simulink model "WriteToServo_test"  (R2014b)
settings: Solver=ode3  StartTime=0.0  StopTime=60  RelTol=1e-3
libraries: ServoCommand x2, BeagleBoneBlackCom x1
settings Model: SimulationMode=external  Creator=Sebastian  LastModifiedBy=Sebastian
settings OptimizationCC: OptimizeModelRefInitCode=on  LifeSpan=1  MaxStackSize=64
settings HardwareCC: ProdLargestAtomicInteger=Long  ProdLargestAtomicFloat=Double  ProdEndianess=LittleEndian  ProdHWDeviceType=ARM Compatible->ARM Cortex
settings RTWCC: SystemTargetFile=ert.tlc  TLCOptions=-aInlineSetEventsForThisBaseRateFcn=TLC_FALSE -aSuppressMultiTaskScheduler=TLC_FALSE  TemplateMakefile=ert_default_tmf  Description=Embedded Coder  ProcessScript=ert_make_rtw_hook  Toolchain=Linaro Toolchain v4.8  BuildConfiguration=Specify
settings CodeAppCC: IgnoreCustomStorageClasses=off

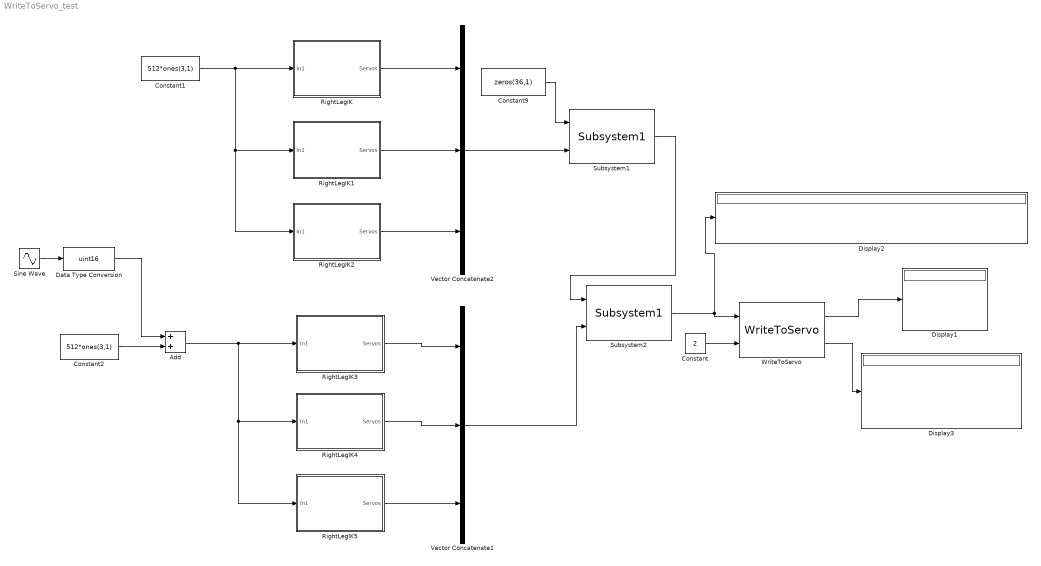
== system WriteToServo_test ==
  Add : Sum
  Constant : Constant  Value=2  OutDataTypeStr=uint8
  Constant1 : Constant  Value=512*ones(3,1)  OutDataTypeStr=uint16  SampleTime=-1
  Constant2 : Constant  Value=512*ones(3,1)  OutDataTypeStr=uint16  SampleTime=-1
  Constant9 : Constant  Value=zeros(36,1)  OutDataTypeStr=uint8  SampleTime=-1
  Data Type Conversion : DataTypeConversion  OutDataTypeStr=uint16
  Display1 : Display
      settings: Format=hex (Stored Integer)
  Display2 : Display
      settings: Format=hex (Stored Integer)
  Display3 : Display
      settings: Format=hex (Stored Integer)
  RightLegIK : Subsystem  TreatAsAtomicUnit=on  RTWFcnName=RightLegIK  mask{ID1=1, ID2=2, ID3=3}
      mask prompts: ID1 "Id servo 1"; ID2 "Id servo 2"; ID3 "Id servo 3"
      settings: RTWFcnNameOpts=User specified
      mask Display: fprintf('ID: %d,%d,%d',ID1,ID2,ID3)
  RightLegIK1 : Subsystem  TreatAsAtomicUnit=on  RTWFcnName=RightLegIK  mask{ID1=4, ID2=5, ID3=6}
      mask prompts: ID1 "Id servo 1"; ID2 "Id servo 2"; ID3 "Id servo 3"
      settings: RTWFcnNameOpts=User specified
      mask Display: fprintf('ID: %d,%d,%d',ID1,ID2,ID3)
  RightLegIK2 : Subsystem  TreatAsAtomicUnit=on  RTWFcnName=RightLegIK  mask{ID1=7, ID2=8, ID3=9}
      mask prompts: ID1 "Id servo 1"; ID2 "Id servo 2"; ID3 "Id servo 3"
      settings: RTWFcnNameOpts=User specified
      mask Display: fprintf('ID: %d,%d,%d',ID1,ID2,ID3)
  RightLegIK3 : Subsystem  TreatAsAtomicUnit=on  RTWFcnName=RightLegIK  mask{ID1=10, ID2=11, ID3=12}
      mask prompts: ID1 "Id servo 1"; ID2 "Id servo 2"; ID3 "Id servo 3"
      settings: RTWFcnNameOpts=User specified
      mask Display: fprintf('ID: %d,%d,%d',ID1,ID2,ID3)
  RightLegIK4 : Subsystem  TreatAsAtomicUnit=on  RTWFcnName=RightLegIK  mask{ID1=13, ID2=14, ID3=15}
      mask prompts: ID1 "Id servo 1"; ID2 "Id servo 2"; ID3 "Id servo 3"
      settings: RTWFcnNameOpts=User specified
      mask Display: fprintf('ID: %d,%d,%d',ID1,ID2,ID3)
  RightLegIK5 : Subsystem  TreatAsAtomicUnit=on  RTWFcnName=RightLegIK  mask{ID1=16, ID2=17, ID3=18}
      mask prompts: ID1 "Id servo 1"; ID2 "Id servo 2"; ID3 "Id servo 3"
      settings: RTWFcnNameOpts=User specified
      mask Display: fprintf('ID: %d,%d,%d',ID1,ID2,ID3)
  Sine Wave : Sin  Amplitude=100  Frequency=3  SampleTime=0.05
  Subsystem1 : ServoCommand/Subsystem1
  Subsystem2 : ServoCommand/Subsystem1
  Vector Concatenate1 : Concatenate  NumInputs=3  ConcatenateDimension=2
  Vector Concatenate2 : Concatenate  NumInputs=3  ConcatenateDimension=2
  WriteToServo : BeagleBoneBlackCom/WriteToServo
  wires:
  RightLegIK1/1(Servos) -> Vector Concatenate2/2
  RightLegIK2/1(Servos) -> Vector Concatenate2/3
  Constant1/1 -> RightLegIK2/1(In1), RightLegIK1/1(In1), RightLegIK/1(In1)
  RightLegIK3/1(Servos) -> Vector Concatenate1/1
  RightLegIK4/1(Servos) -> Vector Concatenate1/2
  RightLegIK5/1(Servos) -> Vector Concatenate1/3
  Add/1 -> RightLegIK5/1(In1), RightLegIK4/1(In1), RightLegIK3/1(In1)
  Sine Wave/1 -> Data Type Conversion/1
  Constant2/1 -> Add/2
  Data Type Conversion/1 -> Add/1
  Constant/1 -> WriteToServo/2
  WriteToServo/2 -> Display3/1
  WriteToServo/1 -> Display1/1
  Vector Concatenate1/1 -> Subsystem2/2
  Subsystem2/1 -> WriteToServo/1, Display2/1
  Subsystem1/1 -> Subsystem2/1
  Vector Concatenate2/1 -> Subsystem1/2
  Constant9/1 -> Subsystem1/1
  RightLegIK/1(Servos) -> Vector Concatenate2/1

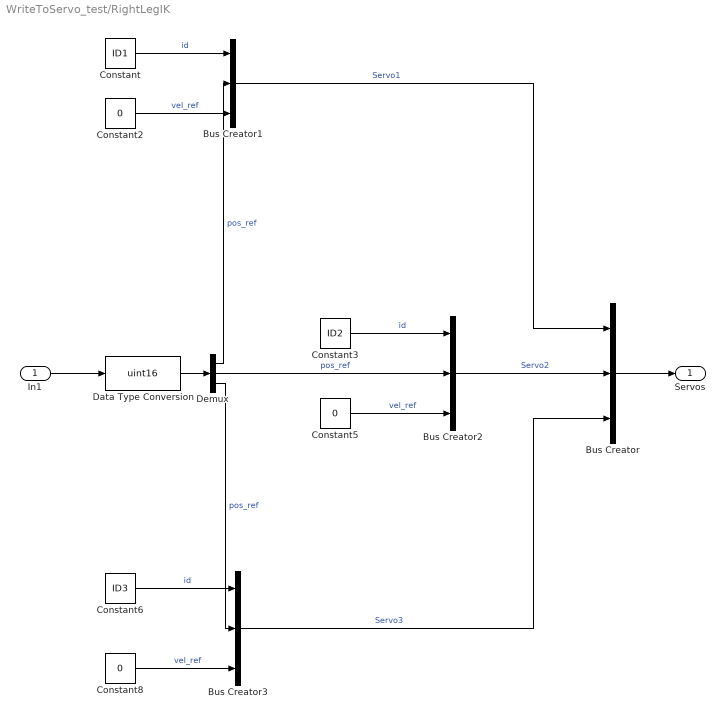
== system WriteToServo_test/RightLegIK ==
  In1 : Inport
  Bus Creator : BusCreator  Inputs=3  OutDataTypeStr=Bus: Leg_ref  NonVirtualBus=on
      settings: InheritFromInputs=off
  Bus Creator1 : BusCreator  Inputs=3  OutDataTypeStr=Bus: Servo  NonVirtualBus=on
      settings: InheritFromInputs=off
  Bus Creator2 : BusCreator  Inputs=3  OutDataTypeStr=Bus: Servo  NonVirtualBus=on
      settings: InheritFromInputs=off
  Bus Creator3 : BusCreator  Inputs=3  OutDataTypeStr=Bus: Servo  NonVirtualBus=on
      settings: InheritFromInputs=off
  Constant : Constant  Value=ID1  OutDataTypeStr=uint8  SampleTime=-1
  Constant2 : Constant  Value=0  OutDataTypeStr=uint16  SampleTime=-1
  Constant3 : Constant  Value=ID2  OutDataTypeStr=uint8  SampleTime=-1
  Constant5 : Constant  Value=0  OutDataTypeStr=uint16  SampleTime=-1
  Constant6 : Constant  Value=ID3  OutDataTypeStr=uint8  SampleTime=-1
  Constant8 : Constant  Value=0  OutDataTypeStr=uint16  SampleTime=-1
  Data Type Conversion : DataTypeConversion  OutDataTypeStr=uint16
  Demux : Demux  Outputs=3
  Servos : Outport  OutDataTypeStr=Bus: Leg_ref  PortDimensions=3
  wires:
  Constant8/1 -> Bus Creator3/3  "vel_ref"
  Constant5/1 -> Bus Creator2/3  "vel_ref"
  Constant2/1 -> Bus Creator1/3  "vel_ref"
  Data Type Conversion/1 -> Demux/1
  Demux/2 -> Bus Creator2/2  "pos_ref"
  Demux/3 -> Bus Creator3/2  "pos_ref"
  Constant6/1 -> Bus Creator3/1  "id"
  Constant3/1 -> Bus Creator2/1  "id"
  Bus Creator3/1 -> Bus Creator/3  "Servo3"
  Demux/1 -> Bus Creator1/2  "pos_ref"
  Constant/1 -> Bus Creator1/1  "id"
  Bus Creator2/1 -> Bus Creator/2  "Servo2"
  Bus Creator1/1 -> Bus Creator/1  "Servo1"
  Bus Creator/1 -> Servos/1
  In1/1 -> Data Type Conversion/1

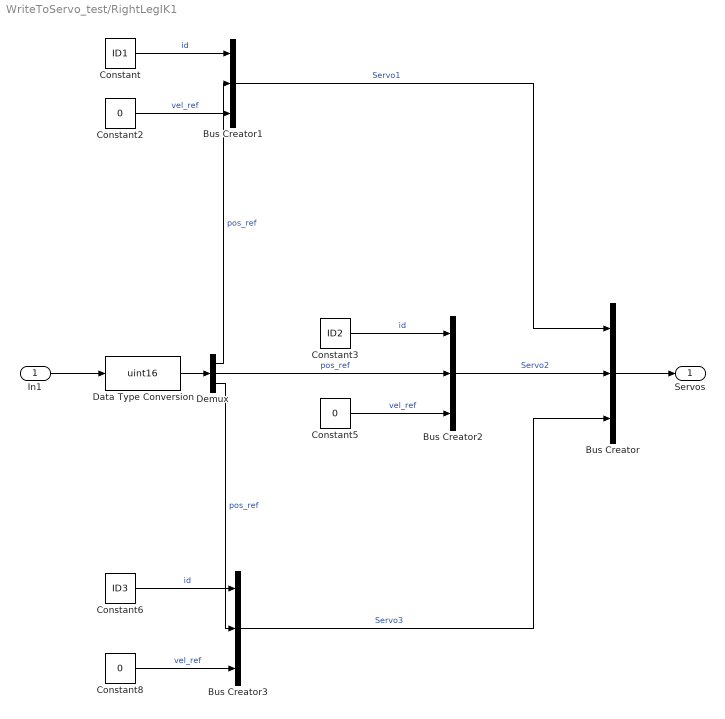
== system WriteToServo_test/RightLegIK1 ==
  In1 : Inport
  Bus Creator : BusCreator  Inputs=3  OutDataTypeStr=Bus: Leg_ref  NonVirtualBus=on
      settings: InheritFromInputs=off
  Bus Creator1 : BusCreator  Inputs=3  OutDataTypeStr=Bus: Servo  NonVirtualBus=on
      settings: InheritFromInputs=off
  Bus Creator2 : BusCreator  Inputs=3  OutDataTypeStr=Bus: Servo  NonVirtualBus=on
      settings: InheritFromInputs=off
  Bus Creator3 : BusCreator  Inputs=3  OutDataTypeStr=Bus: Servo  NonVirtualBus=on
      settings: InheritFromInputs=off
  Constant : Constant  Value=ID1  OutDataTypeStr=uint8  SampleTime=-1
  Constant2 : Constant  Value=0  OutDataTypeStr=uint16  SampleTime=-1
  Constant3 : Constant  Value=ID2  OutDataTypeStr=uint8  SampleTime=-1
  Constant5 : Constant  Value=0  OutDataTypeStr=uint16  SampleTime=-1
  Constant6 : Constant  Value=ID3  OutDataTypeStr=uint8  SampleTime=-1
  Constant8 : Constant  Value=0  OutDataTypeStr=uint16  SampleTime=-1
  Data Type Conversion : DataTypeConversion  OutDataTypeStr=uint16
  Demux : Demux  Outputs=3
  Servos : Outport  OutDataTypeStr=Bus: Leg_ref  PortDimensions=3
  wires:
  Constant8/1 -> Bus Creator3/3  "vel_ref"
  Constant5/1 -> Bus Creator2/3  "vel_ref"
  Constant2/1 -> Bus Creator1/3  "vel_ref"
  Data Type Conversion/1 -> Demux/1
  Demux/2 -> Bus Creator2/2  "pos_ref"
  Demux/3 -> Bus Creator3/2  "pos_ref"
  Constant6/1 -> Bus Creator3/1  "id"
  Constant3/1 -> Bus Creator2/1  "id"
  Bus Creator3/1 -> Bus Creator/3  "Servo3"
  Demux/1 -> Bus Creator1/2  "pos_ref"
  Constant/1 -> Bus Creator1/1  "id"
  Bus Creator2/1 -> Bus Creator/2  "Servo2"
  Bus Creator1/1 -> Bus Creator/1  "Servo1"
  Bus Creator/1 -> Servos/1
  In1/1 -> Data Type Conversion/1

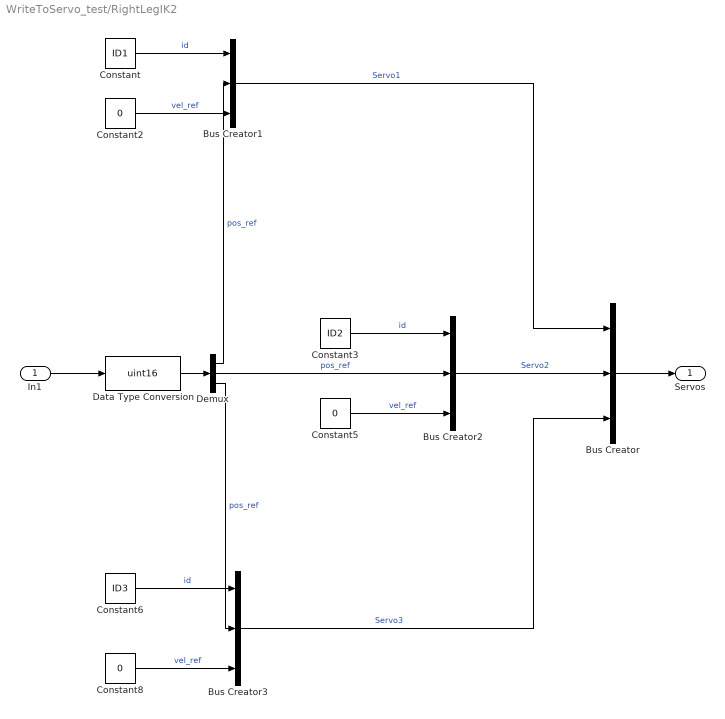
== system WriteToServo_test/RightLegIK2 ==
  In1 : Inport
  Bus Creator : BusCreator  Inputs=3  OutDataTypeStr=Bus: Leg_ref  NonVirtualBus=on
      settings: InheritFromInputs=off
  Bus Creator1 : BusCreator  Inputs=3  OutDataTypeStr=Bus: Servo  NonVirtualBus=on
      settings: InheritFromInputs=off
  Bus Creator2 : BusCreator  Inputs=3  OutDataTypeStr=Bus: Servo  NonVirtualBus=on
      settings: InheritFromInputs=off
  Bus Creator3 : BusCreator  Inputs=3  OutDataTypeStr=Bus: Servo  NonVirtualBus=on
      settings: InheritFromInputs=off
  Constant : Constant  Value=ID1  OutDataTypeStr=uint8  SampleTime=-1
  Constant2 : Constant  Value=0  OutDataTypeStr=uint16  SampleTime=-1
  Constant3 : Constant  Value=ID2  OutDataTypeStr=uint8  SampleTime=-1
  Constant5 : Constant  Value=0  OutDataTypeStr=uint16  SampleTime=-1
  Constant6 : Constant  Value=ID3  OutDataTypeStr=uint8  SampleTime=-1
  Constant8 : Constant  Value=0  OutDataTypeStr=uint16  SampleTime=-1
  Data Type Conversion : DataTypeConversion  OutDataTypeStr=uint16
  Demux : Demux  Outputs=3
  Servos : Outport  OutDataTypeStr=Bus: Leg_ref  PortDimensions=3
  wires:
  Constant8/1 -> Bus Creator3/3  "vel_ref"
  Constant5/1 -> Bus Creator2/3  "vel_ref"
  Constant2/1 -> Bus Creator1/3  "vel_ref"
  Data Type Conversion/1 -> Demux/1
  Demux/2 -> Bus Creator2/2  "pos_ref"
  Demux/3 -> Bus Creator3/2  "pos_ref"
  Constant6/1 -> Bus Creator3/1  "id"
  Constant3/1 -> Bus Creator2/1  "id"
  Bus Creator3/1 -> Bus Creator/3  "Servo3"
  Demux/1 -> Bus Creator1/2  "pos_ref"
  Constant/1 -> Bus Creator1/1  "id"
  Bus Creator2/1 -> Bus Creator/2  "Servo2"
  Bus Creator1/1 -> Bus Creator/1  "Servo1"
  Bus Creator/1 -> Servos/1
  In1/1 -> Data Type Conversion/1

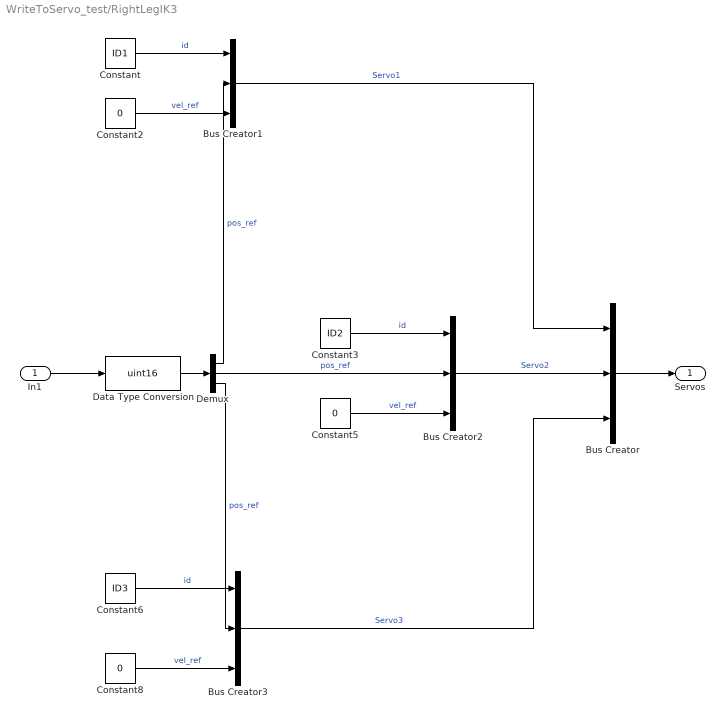
== system WriteToServo_test/RightLegIK3 ==
  In1 : Inport
  Bus Creator : BusCreator  Inputs=3  OutDataTypeStr=Bus: Leg_ref  NonVirtualBus=on
      settings: InheritFromInputs=off
  Bus Creator1 : BusCreator  Inputs=3  OutDataTypeStr=Bus: Servo  NonVirtualBus=on
      settings: InheritFromInputs=off
  Bus Creator2 : BusCreator  Inputs=3  OutDataTypeStr=Bus: Servo  NonVirtualBus=on
      settings: InheritFromInputs=off
  Bus Creator3 : BusCreator  Inputs=3  OutDataTypeStr=Bus: Servo  NonVirtualBus=on
      settings: InheritFromInputs=off
  Constant : Constant  Value=ID1  OutDataTypeStr=uint8  SampleTime=-1
  Constant2 : Constant  Value=0  OutDataTypeStr=uint16  SampleTime=-1
  Constant3 : Constant  Value=ID2  OutDataTypeStr=uint8  SampleTime=-1
  Constant5 : Constant  Value=0  OutDataTypeStr=uint16  SampleTime=-1
  Constant6 : Constant  Value=ID3  OutDataTypeStr=uint8  SampleTime=-1
  Constant8 : Constant  Value=0  OutDataTypeStr=uint16  SampleTime=-1
  Data Type Conversion : DataTypeConversion  OutDataTypeStr=uint16
  Demux : Demux  Outputs=3
  Servos : Outport  OutDataTypeStr=Bus: Leg_ref  PortDimensions=3
  wires:
  Constant8/1 -> Bus Creator3/3  "vel_ref"
  Constant5/1 -> Bus Creator2/3  "vel_ref"
  Constant2/1 -> Bus Creator1/3  "vel_ref"
  Data Type Conversion/1 -> Demux/1
  Demux/2 -> Bus Creator2/2  "pos_ref"
  Demux/3 -> Bus Creator3/2  "pos_ref"
  Constant6/1 -> Bus Creator3/1  "id"
  Constant3/1 -> Bus Creator2/1  "id"
  Bus Creator3/1 -> Bus Creator/3  "Servo3"
  Demux/1 -> Bus Creator1/2  "pos_ref"
  Constant/1 -> Bus Creator1/1  "id"
  Bus Creator2/1 -> Bus Creator/2  "Servo2"
  Bus Creator1/1 -> Bus Creator/1  "Servo1"
  Bus Creator/1 -> Servos/1
  In1/1 -> Data Type Conversion/1

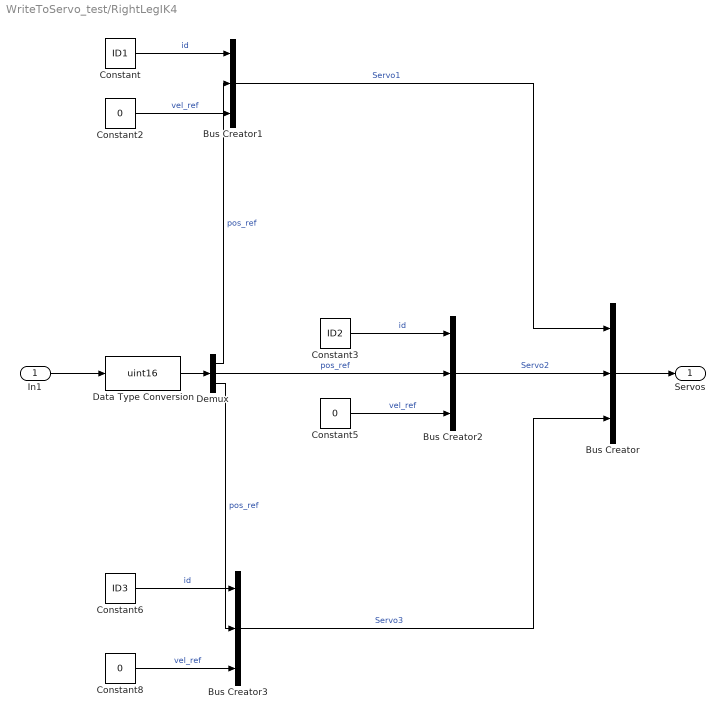
== system WriteToServo_test/RightLegIK4 ==
  In1 : Inport
  Bus Creator : BusCreator  Inputs=3  OutDataTypeStr=Bus: Leg_ref  NonVirtualBus=on
      settings: InheritFromInputs=off
  Bus Creator1 : BusCreator  Inputs=3  OutDataTypeStr=Bus: Servo  NonVirtualBus=on
      settings: InheritFromInputs=off
  Bus Creator2 : BusCreator  Inputs=3  OutDataTypeStr=Bus: Servo  NonVirtualBus=on
      settings: InheritFromInputs=off
  Bus Creator3 : BusCreator  Inputs=3  OutDataTypeStr=Bus: Servo  NonVirtualBus=on
      settings: InheritFromInputs=off
  Constant : Constant  Value=ID1  OutDataTypeStr=uint8  SampleTime=-1
  Constant2 : Constant  Value=0  OutDataTypeStr=uint16  SampleTime=-1
  Constant3 : Constant  Value=ID2  OutDataTypeStr=uint8  SampleTime=-1
  Constant5 : Constant  Value=0  OutDataTypeStr=uint16  SampleTime=-1
  Constant6 : Constant  Value=ID3  OutDataTypeStr=uint8  SampleTime=-1
  Constant8 : Constant  Value=0  OutDataTypeStr=uint16  SampleTime=-1
  Data Type Conversion : DataTypeConversion  OutDataTypeStr=uint16
  Demux : Demux  Outputs=3
  Servos : Outport  OutDataTypeStr=Bus: Leg_ref  PortDimensions=3
  wires:
  Constant8/1 -> Bus Creator3/3  "vel_ref"
  Constant5/1 -> Bus Creator2/3  "vel_ref"
  Constant2/1 -> Bus Creator1/3  "vel_ref"
  Data Type Conversion/1 -> Demux/1
  Demux/2 -> Bus Creator2/2  "pos_ref"
  Demux/3 -> Bus Creator3/2  "pos_ref"
  Constant6/1 -> Bus Creator3/1  "id"
  Constant3/1 -> Bus Creator2/1  "id"
  Bus Creator3/1 -> Bus Creator/3  "Servo3"
  Demux/1 -> Bus Creator1/2  "pos_ref"
  Constant/1 -> Bus Creator1/1  "id"
  Bus Creator2/1 -> Bus Creator/2  "Servo2"
  Bus Creator1/1 -> Bus Creator/1  "Servo1"
  Bus Creator/1 -> Servos/1
  In1/1 -> Data Type Conversion/1

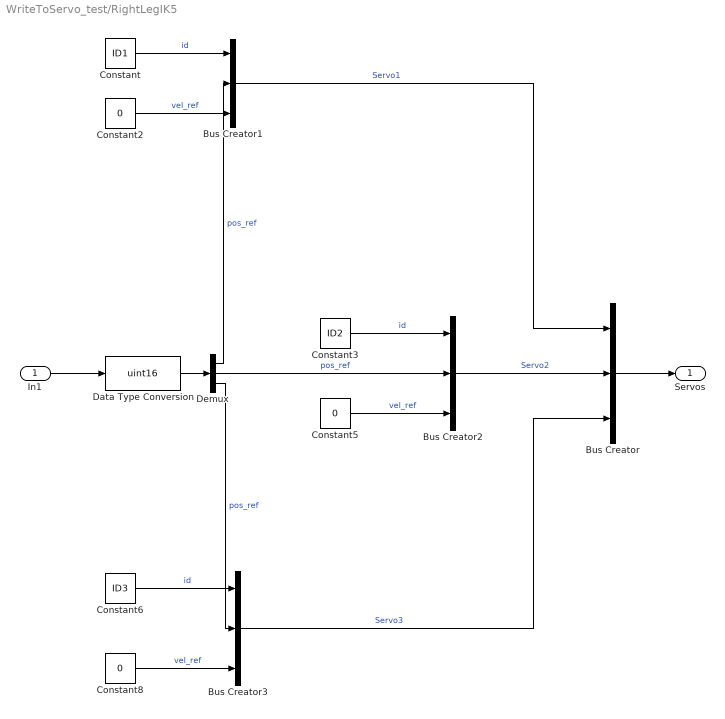
== system WriteToServo_test/RightLegIK5 ==
  In1 : Inport
  Bus Creator : BusCreator  Inputs=3  OutDataTypeStr=Bus: Leg_ref  NonVirtualBus=on
      settings: InheritFromInputs=off
  Bus Creator1 : BusCreator  Inputs=3  OutDataTypeStr=Bus: Servo  NonVirtualBus=on
      settings: InheritFromInputs=off
  Bus Creator2 : BusCreator  Inputs=3  OutDataTypeStr=Bus: Servo  NonVirtualBus=on
      settings: InheritFromInputs=off
  Bus Creator3 : BusCreator  Inputs=3  OutDataTypeStr=Bus: Servo  NonVirtualBus=on
      settings: InheritFromInputs=off
  Constant : Constant  Value=ID1  OutDataTypeStr=uint8  SampleTime=-1
  Constant2 : Constant  Value=0  OutDataTypeStr=uint16  SampleTime=-1
  Constant3 : Constant  Value=ID2  OutDataTypeStr=uint8  SampleTime=-1
  Constant5 : Constant  Value=0  OutDataTypeStr=uint16  SampleTime=-1
  Constant6 : Constant  Value=ID3  OutDataTypeStr=uint8  SampleTime=-1
  Constant8 : Constant  Value=0  OutDataTypeStr=uint16  SampleTime=-1
  Data Type Conversion : DataTypeConversion  OutDataTypeStr=uint16
  Demux : Demux  Outputs=3
  Servos : Outport  OutDataTypeStr=Bus: Leg_ref  PortDimensions=3
  wires:
  Constant8/1 -> Bus Creator3/3  "vel_ref"
  Constant5/1 -> Bus Creator2/3  "vel_ref"
  Constant2/1 -> Bus Creator1/3  "vel_ref"
  Data Type Conversion/1 -> Demux/1
  Demux/2 -> Bus Creator2/2  "pos_ref"
  Demux/3 -> Bus Creator3/2  "pos_ref"
  Constant6/1 -> Bus Creator3/1  "id"
  Constant3/1 -> Bus Creator2/1  "id"
  Bus Creator3/1 -> Bus Creator/3  "Servo3"
  Demux/1 -> Bus Creator1/2  "pos_ref"
  Constant/1 -> Bus Creator1/1  "id"
  Bus Creator2/1 -> Bus Creator/2  "Servo2"
  Bus Creator1/1 -> Bus Creator/1  "Servo1"
  Bus Creator/1 -> Servos/1
  In1/1 -> Data Type Conversion/1
